simulink model "sedemo_timrecresample"  (Simulink 7.5)
settings: Solver=ode45  StartTime=0.0  StopTime=inf  MaxStep=1/(10*D*Fsymbol)  RelTol=1e-3
PreLoadFcn:
  | Fsymbol=1e6;
  | D=8;  % decimation / interpolation
  | Fdelay = 5;  % rrc filter delay
  | Alpha = 0.25;  % excess BW
  | rrc_coef=rcosine(1,D,'fir/sqrt',Alpha,Fdelay);
  | rrc_coef=rrc_coef/sum(rrc_coef);
  | Carrier_Freq = 21.4e6;
  | b3 = [1/6 -1/2  1/2 -1/6];
  | b2 = [1/2 -1    1/2  0];
  | b1 = [1/3  1/2 -1    1/6];
  | b0 = [0    1    0    0];
undefined symbols (not defined in the file or in its folder): dfilt, j, magnitude
libraries: dspsigops x29, simulink x13, dsparch4 x8, dspsrcs4 x4, dspbuff3 x2, simeventsinfo x1, simeventstranslate1 x1, dspmlti4 x1, commsink2 x1
CloseFcn:
  | clear Fsymbol D Fdelay Alpha rrc_coef Carrier_Freq b0 b1 b2 b3;
settings Model: Creator=The MathWorks Inc.  ExtModeAutoUpdateStatusClock=off
settings DataIOCC: SaveOutput=off  SignalLogging=off  SaveTime=off
settings OptimizationCC: InitFltsAndDblsToZero=on  EfficientMapNaN2IntZero=off
settings DebuggingCC: SignalResolutionControl=TryResolveAllWithWarning  MultiTaskDSMMsg=warning  MultiTaskCondExecSysMsg=none  SigSpecEnsureSampleTimeMsg=none  StrictBusMsg=None
settings RTWCC: IncludeERTFirstTime=on
settings SimEventsCC: propDiagAttribOutput=1  propDiagFcnCallOutput=1  propDiagStatOutput=0

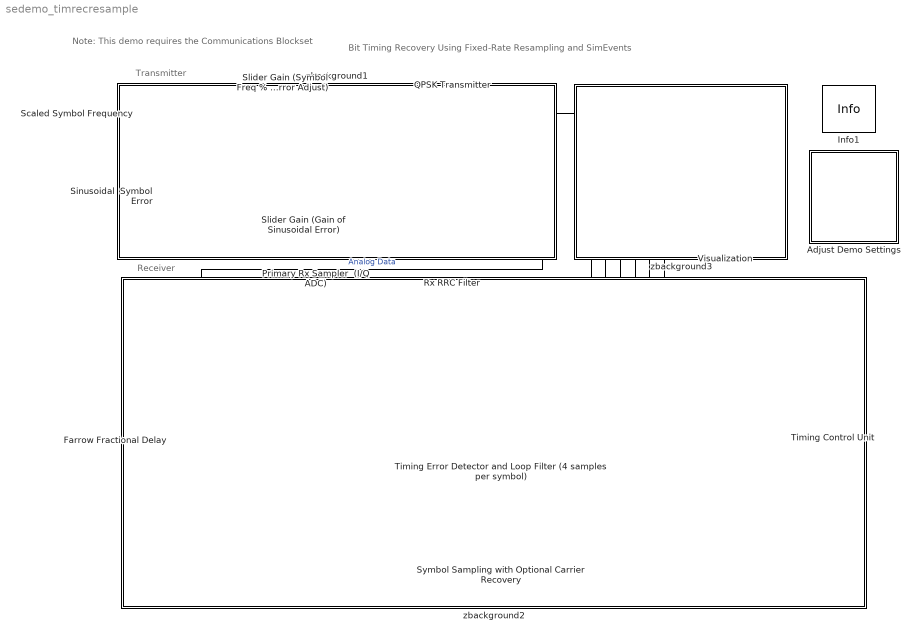
== system sedemo_timrecresample ==
  note: Bit Timing Recovery Using Fixed-Rate
      | Resampling and SimEvents
  note: Transmitter
  note: Receiver
  note: Note: This demo requires the
      | Communications Blockset
  Adjust Demo Settings : Subsystem  mask(Timing Recovery Demo Settings){enableTCU=on}
      mask prompts: enableTCU "Enable timing control"
      mask help:
      | Click on the 'Enable timing control' checkbox while the demo is running to enable and disable the timing control for the receiver.
      |
      | Note that you can also change the slider gain values for Symbol Frequency Percent Error and Gain of Sinusoidal Error while the demo is running.
      mask init:
      | set_param([bdroot '/Timing Control Unit/TCU_ON'],'Value',num2str(enableTCU));
      mask Display: disp('Timing\nRecovery\nDemo\nSettings');
  "Farrow Fractional Delay " : Subsystem
  Info1 : simeventsinfo/Info  SystemSampleTime=-1
  Primary Rx Sampler  (I/Q ADC) : ZeroOrderHold  SampleTime=1/(D*Fsymbol)
  QPSK Transmitter : Subsystem
  Rx RRC Filter : dspmlti4/FIR Decimation  DialogController=dspdialog.FIRDecimation  DialogControllerArgs=DataTag6  h=rrc_coef  D=2  filtStruct=Direct form  framing=Maintain input frame size  inputOffset=0  outputBufInitCond=0  roundingMode=Floor  overflowMode=off  FilterSource=Specify via dialog  FilterObject=Hm_firdecim
  Scaled Symbol Frequency : Constant  Value=(D*Fsymbol) / 100  OutDataType=sfix(16)  OutScaling=2^0
  Sinusoidal  Symbol Error : Sin  Amplitude=(D*Fsymbol) / 100  Bias=0  Frequency=(Fsymbol)*2*pi/1000  Phase=0  Samples=10  SampleTime=1e-5  Offset=0
  Slider Gain (Gain of Sinusoidal Error) : simulink/Math Operations/Slider Gain  SystemSampleTime=-1  low=0  gain=0.1  high=0.2
  Slider Gain (Symbol Freq % Error Adjust) : simulink/Math Operations/Slider Gain  SystemSampleTime=-1  low=-0.2  gain=0.02  high=0.2
  Symbol Sampling with Optional Carrier Recovery : Subsystem
  Timing Control Unit : Subsystem
  Timing Error Detector and Loop Filter (4 samples per symbol) : Subsystem
  Visualization : Subsystem
  zbackground1 : Subsystem
      mask Display: disp('')
  zbackground2 : Subsystem
      mask Display: disp('')
  zbackground3 : Subsystem
      mask Display: disp('')
  wires:
  Scaled Symbol Frequency/1 -> Slider Gain (Symbol Freq % Error Adjust)/1
  Slider Gain (Symbol Freq % Error Adjust)/1 -> QPSK Transmitter/1(Constant Sym Err)
  Slider Gain (Gain of Sinusoidal Error)/1 -> QPSK Transmitter/2(Sinusoidal Sym Err)
  Sinusoidal  Symbol Error/1 -> Slider Gain (Gain of Sinusoidal Error)/1
  QPSK Transmitter/1(Tx Sym Clk) -> Visualization/1(Tx Sym Clk)
  QPSK Transmitter/2(Tx Data) -> Primary Rx Sampler  (I/Q ADC)/1  "Analog Data"
  "Farrow Fractional Delay "/1(X(n-(1-u))) -> Timing Error Detector and Loop Filter (4 samples per symbol)/2(I/Q In), Symbol Sampling with Optional Carrier Recovery/2(Data)
  Primary Rx Sampler  (I/Q ADC)/1 -> Rx RRC Filter/1
  Rx RRC Filter/1 -> "Farrow Fractional Delay "/1(X(n))
  Timing Control Unit/1(Symbol Clk) -> Timing Error Detector and Loop Filter (4 samples per symbol)/1(Symbol Clk), Symbol Sampling with Optional Carrier Recovery/1(Symbol Clk), Visualization/2(Rx Rec Sym Clk)
  Timing Control Unit/2(Delay Ctrl) -> "Farrow Fractional Delay "/2(u), Visualization/7(Frac Dly Ctrl)
  Timing Error Detector and Loop Filter (4 samples per symbol)/2(Timing Ctrl) -> Timing Control Unit/1(Ctrl In), Visualization/4(TCU Ctrl)
  Timing Error Detector and Loop Filter (4 samples per symbol)/1(Timing Err) -> Visualization/3(Timing Err)
  Symbol Sampling with Optional Carrier Recovery/1(Delayed Clk) -> Visualization/5(Delayed Clk)
  Symbol Sampling with Optional Carrier Recovery/2(Symbol) -> Visualization/6(Rx Symbol)

== system sedemo_timrecresample/Adjust Demo Settings ==

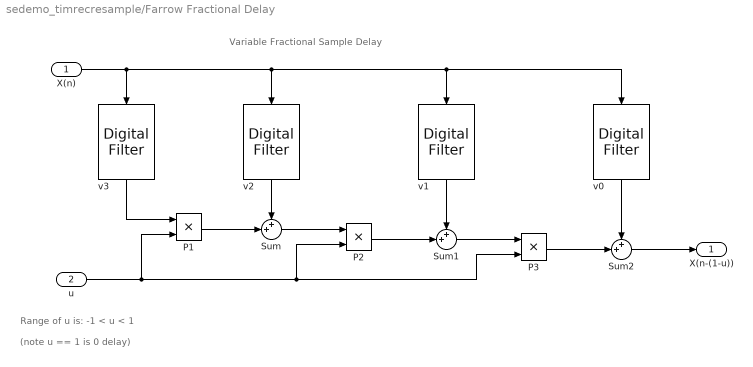
== system sedemo_timrecresample/Farrow Fractional Delay  ==
  note: Range of u is: -1 < u < 1
  note: Variable Fractional Sample Delay
  note: (note u == 1 is 0 delay)
  X(n) : Inport  OutDataType=sfix(16)  OutScaling=2^0
  u : Inport  Port=2  OutDataType=sfix(16)  OutScaling=2^0
  P1 : Product  OutDataType=sfix(16)  OutScaling=2^0  SaturateOnIntegerOverflow=on  OutDataTypeStr=Inherit: Same as first input
  P2 : Product  OutDataType=sfix(16)  OutScaling=2^0  SaturateOnIntegerOverflow=on  OutDataTypeStr=Inherit: Same as first input
  P3 : Product  OutDataType=sfix(16)  OutScaling=2^0  SaturateOnIntegerOverflow=on  OutDataTypeStr=Inherit: Same as first input
  Sum : Sum  Inputs=++|  OutDataType=sfix(16)  OutScaling=2^0  SaturateOnIntegerOverflow=on
  Sum1 : Sum  Inputs=++|  OutDataType=sfix(16)  OutScaling=2^0  SaturateOnIntegerOverflow=on
  Sum2 : Sum  Inputs=++|  OutDataType=sfix(16)  OutScaling=2^0  SaturateOnIntegerOverflow=on
  v0 : dsparch4/Digital Filter  DialogController=dspdialog.DigitalFilter  DialogControllerArgs=DataTag0  TypePopup=FIR (all zeros)  IIRFiltStruct=Direct form II transposed  AllPoleFiltStruct=Direct form  FIRFiltStruct=Direct form  CoeffSource=Specify via dialog  NumCoeffs=b0  DenCoeffs=[1 0.1]  BiQuadCoeffs=[1 0.3 0.4 1 0.1 0.2]  LatticeCoeffs=[0.2 0.4]  denIgnore=on  FiltPerSampPopup=One filter per frame  IC=0  ICnum=0  ICden=0  roundingMode=Floor  overflowMode=off  ScaleValues=1  scaleValueFracLength=14  stageInFracLength=15  stageOutFracLength=15  FilterSource=Specify via dialog  dfiltObjectName=dfilt.dffir([1 2 1])
  v1 : dsparch4/Digital Filter  DialogController=dspdialog.DigitalFilter  DialogControllerArgs=DataTag1  TypePopup=FIR (all zeros)  IIRFiltStruct=Direct form II transposed  AllPoleFiltStruct=Direct form  FIRFiltStruct=Direct form  CoeffSource=Specify via dialog  NumCoeffs=b1  DenCoeffs=[1 0.1]  BiQuadCoeffs=[1 0.3 0.4 1 0.1 0.2]  LatticeCoeffs=[0.2 0.4]  denIgnore=on  FiltPerSampPopup=One filter per frame  IC=0  ICnum=0  ICden=0  roundingMode=Floor  overflowMode=off  ScaleValues=1  scaleValueFracLength=14  stageInFracLength=15  stageOutFracLength=15  FilterSource=Specify via dialog  dfiltObjectName=dfilt.dffir([1 2 1])
  v2 : dsparch4/Digital Filter  DialogController=dspdialog.DigitalFilter  DialogControllerArgs=DataTag2  TypePopup=FIR (all zeros)  IIRFiltStruct=Direct form II transposed  AllPoleFiltStruct=Direct form  FIRFiltStruct=Direct form  CoeffSource=Specify via dialog  NumCoeffs=b2  DenCoeffs=[1 0.1]  BiQuadCoeffs=[1 0.3 0.4 1 0.1 0.2]  LatticeCoeffs=[0.2 0.4]  denIgnore=on  FiltPerSampPopup=One filter per frame  IC=0  ICnum=0  ICden=0  roundingMode=Floor  overflowMode=off  ScaleValues=1  scaleValueFracLength=14  stageInFracLength=15  stageOutFracLength=15  FilterSource=Specify via dialog  dfiltObjectName=dfilt.dffir([1 2 1])
  v3 : dsparch4/Digital Filter  DialogController=dspdialog.DigitalFilter  DialogControllerArgs=DataTag3  TypePopup=FIR (all zeros)  IIRFiltStruct=Direct form II transposed  AllPoleFiltStruct=Direct form  FIRFiltStruct=Direct form  CoeffSource=Specify via dialog  NumCoeffs=b3  DenCoeffs=[1 0.1]  BiQuadCoeffs=[1 0.3 0.4 1 0.1 0.2]  LatticeCoeffs=[0.2 0.4]  denIgnore=on  FiltPerSampPopup=One filter per frame  IC=0  ICnum=0  ICden=0  roundingMode=Floor  overflowMode=off  ScaleValues=1  scaleValueFracLength=14  stageInFracLength=15  stageOutFracLength=15  FilterSource=Specify via dialog  dfiltObjectName=dfilt.dffir([1 2 1])
  X(n-(1-u)) : Outport  OutDataType=sfix(16)  OutScaling=2^0
  wires:
  Sum2/1 -> X(n-(1-u))/1
  u/1 -> P3/2, P2/2, P1/2
  X(n)/1 -> v3/1, v2/1, v1/1, v0/1
  v0/1 -> Sum2/1
  v1/1 -> Sum1/1
  v2/1 -> Sum/1
  v3/1 -> P1/1
  P1/1 -> Sum/2
  Sum/1 -> P2/1
  P2/1 -> Sum1/2
  Sum1/1 -> P3/1
  P3/1 -> Sum2/2

== system sedemo_timrecresample/QPSK Transmitter ==
  note: 1/Ts=D*Fsymbol
  Constant Sym Err : Inport  OutDataType=sfix(16)  OutScaling=2^0
  Sinusoidal Sym Err : Inport  Port=2  OutDataType=sfix(16)  OutScaling=2^0
  Carrier Offset and Conversion to Continuous Time : Subsystem
  DES Voltage Controlled  Sample Rate : Subsystem
  Variable Rate Symbol Generator : Subsystem  TreatAsAtomicUnit=on
      settings: PropExecContextOutsideSubsystem=on
  Tx Sym Clk : Outport  OutDataType=sfix(16)  OutScaling=2^0
  Tx Data : Outport  Port=2  OutDataType=sfix(16)  OutScaling=2^0
  wires:
  Variable Rate Symbol Generator/1(RRC'd Symbols) -> Carrier Offset and Conversion to Continuous Time/1(Data)
  Carrier Offset and Conversion to Continuous Time/1(I/Q Out) -> Tx Data/1  "Baseband Continuous-Time Data"
  Sinusoidal Sym Err/1 -> DES Voltage Controlled  Sample Rate/2(Sinusoidal Error)
  Constant Sym Err/1 -> DES Voltage Controlled  Sample Rate/1(Constant Error)
  Variable Rate Symbol Generator/2(Symbol Clk) -> Tx Sym Clk/1  "Symbol Clock"
  DES Voltage Controlled  Sample Rate/1(Out1) -> Variable Rate Symbol Generator/Trigger

== system sedemo_timrecresample/Symbol Sampling with Optional Carrier Recovery ==
  note: Subsequent processing (demodulation, error correction, symbol to bit mapping, etc.)
      | may be placed inside the Symbol Sampler block.
  Symbol Clk : Inport  OutDataType=sfix(16)  OutScaling=2^0
  Data : Inport  Port=2  OutDataType=sfix(16)  OutScaling=2^0
  Carrier_Rec_ON : Constant  Value=0  OutDataTypeMode=boolean  OutDataType=sfix(16)  OutScaling=2^0  OutDataTypeStr=boolean
  Delay : dspsigops/Delay  dly_unit=Samples  delay=2  ic_detail=off  dif_ic_for_ch=off  dif_ic_for_dly=off  ic=0  reset_popup=None
  Symbol Sampler : Subsystem  TreatAsAtomicUnit=on
  Delayed Clk : Outport  OutDataType=sfix(16)  OutScaling=2^0
  Symbol : Outport  Port=2  OutDataType=sfix(16)  OutScaling=2^0
  wires:
  Delay/1 -> Delayed Clk/1, Symbol Sampler/Enable
  Symbol Clk/1 -> Delay/1
  Data/1 -> Symbol Sampler/1(In1)
  Symbol Sampler/1(Out1) -> Symbol/1
  Carrier_Rec_ON/1 -> Symbol Sampler/2(Carrier Recovery ON)

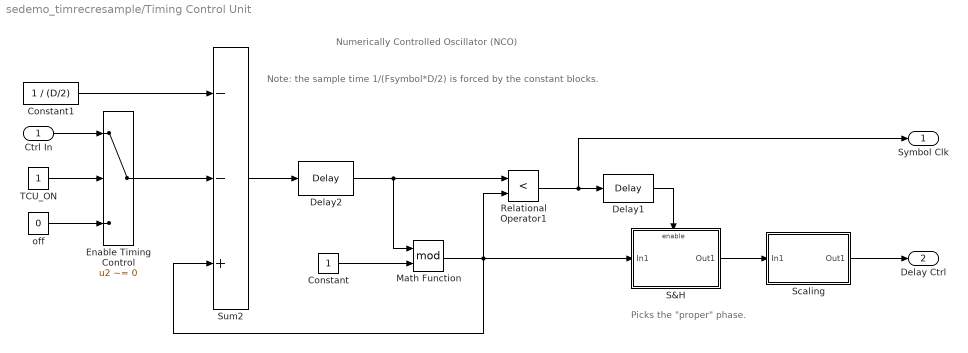
== system sedemo_timrecresample/Timing Control Unit ==
  note: Note:  the sample time 1/(Fsymbol*D/2)
      | is forced by the constant blocks.
  note: Numerically Controlled Oscillator (NCO)
  note: Picks the "proper" phase.
  Ctrl In : Inport  OutDataType=sfix(16)  OutScaling=2^0
  Constant : Constant  OutDataType=sfix(16)  OutScaling=2^0  OutDataTypeStr=Inherit: Inherit via back propagation  SampleTime=1/(Fsymbol*D/2)
  Constant1 : Constant  Value=1 / (D/2)  OutDataType=sfix(16)  OutScaling=2^0  OutDataTypeStr=Inherit: Inherit via back propagation  SampleTime=1/(Fsymbol*D/2)
  Delay1 : dspsigops/Delay  dly_unit=Samples  delay=1  ic_detail=off  dif_ic_for_ch=off  dif_ic_for_dly=off  ic=0  reset_popup=None
  Delay2 : dspsigops/Delay  dly_unit=Samples  delay=1  ic_detail=on  dif_ic_for_ch=off  dif_ic_for_dly=off  ic=0  reset_popup=None
  Enable Timing Control : Switch  Criteria=u2 ~= 0  OutDataType=sfix(16)  OutScaling=2^0
  Math Function : Math  Operator=mod  OutDataType=sfix(16)  OutScaling=2^0  SaturateOnIntegerOverflow=on
  Relational Operator1 : RelationalOperator  Operator=<  LogicOutDataTypeMode=boolean  LogicDataType=double(64)  OutDataTypeStr=boolean
  "S&H " : Subsystem  TreatAsAtomicUnit=on
  Scaling : Subsystem
  Sum2 : Sum  Inputs=--+  OutDataType=sfix(16)  OutScaling=2^0  SaturateOnIntegerOverflow=on  InputSameDT=on  OutDataTypeStr=Inherit: Same as first input
  TCU_ON : Constant  OutDataTypeMode=boolean  OutDataType=sfix(16)  OutScaling=2^0  OutDataTypeStr=boolean
  off : Constant  Value=0  OutDataType=sfix(16)  OutScaling=2^0
  Symbol Clk : Outport  OutDataType=sfix(16)  OutScaling=2^0
  Delay Ctrl : Outport  Port=2  OutDataType=sfix(16)  OutScaling=2^0
  wires:
  Delay2/1 -> Math Function/1, Relational Operator1/1
  Constant/1 -> Math Function/2
  Sum2/1 -> Delay2/1
  Constant1/1 -> Sum2/1
  Math Function/1 -> Sum2/3, Relational Operator1/2, "S&H "/1(In1)
  Relational Operator1/1 -> Delay1/1, Symbol Clk/1
  Delay1/1 -> "S&H "/Enable
  "S&H "/1(Out1) -> Scaling/1(In1)
  Scaling/1(Out1) -> Delay Ctrl/1
  TCU_ON/1 -> Enable Timing Control/2
  off/1 -> Enable Timing Control/3
  Ctrl In/1 -> Enable Timing Control/1
  Enable Timing Control/1 -> Sum2/2

== system sedemo_timrecresample/Timing Error Detector and Loop Filter (4 samples per symbol) ==
  note: H. Meyer et. al. Digital Communications Receivers, chapter 5.4, pp 291
  Symbol Clk : Inport  OutDataType=sfix(16)  OutScaling=2^0
  I/Q In : Inport  Port=2  OutDataType=sfix(16)  OutScaling=2^0
  Mag Sq + Delays : Subsystem
  Timing Error Detector : Subsystem  TreatAsAtomicUnit=on
  Timing Err : Outport  OutDataType=sfix(16)  OutScaling=2^0
  Timing Ctrl : Outport  Port=2  OutDataType=sfix(16)  OutScaling=2^0
  wires:
  Mag Sq + Delays/1(MagSq(u[n-1])) -> Timing Error Detector/1(In1)
  Mag Sq + Delays/2(MagSq(u[n-3])) -> Timing Error Detector/2(In2)
  Mag Sq + Delays/3(MagSq(u[n-2])) -> Timing Error Detector/3(In3)
  Mag Sq + Delays/4(MagSq(u[n])) -> Timing Error Detector/4(In4)
  I/Q In/1 -> Mag Sq + Delays/1(In1)
  Timing Error Detector/1(Error) -> Timing Err/1
  Timing Error Detector/2(Cntrl) -> Timing Ctrl/1
  Symbol Clk/1 -> Timing Error Detector/Enable

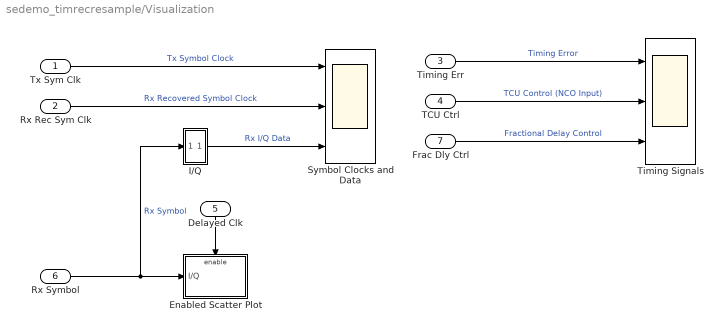
== system sedemo_timrecresample/Visualization ==
  Tx Sym Clk : Inport  OutDataType=sfix(16)  OutScaling=2^0
  Rx Rec Sym Clk : Inport  Port=2  OutDataType=sfix(16)  OutScaling=2^0
  Timing Err : Inport  Port=3  OutDataType=sfix(16)  OutScaling=2^0
  TCU Ctrl : Inport  Port=4  OutDataType=sfix(16)  OutScaling=2^0
  Delayed Clk : Inport  Port=5  OutDataType=sfix(16)  OutScaling=2^0
  Rx Symbol : Inport  Port=6  OutDataType=sfix(16)  OutScaling=2^0
  Frac Dly Ctrl : Inport  Port=7  OutDataType=sfix(16)  OutScaling=2^0
  Enabled Scatter Plot : Subsystem  TreatAsAtomicUnit=on
  I/Q : Subsystem
      mask Display: disp('')
  Symbol Clocks and Data : Scope  NumInputPorts=3
      settings: TimeRange=2e-06  YMin=-0.1~-0.1~-1.5  YMax=1.1~1.1~1.5
  Timing Signals : Scope  NumInputPorts=3
      settings: TimeRange=0.0002  YMin=-0.2~-0.001~-0.1  YMax=0.2~0.001~1.1  MaxDataPoints=50000
  wires:
  Rx Symbol/1 -> I/Q/1(cmplx), Enabled Scatter Plot/1(I/Q)  "Rx Symbol"
  I/Q/1(2x real) -> Symbol Clocks and Data/3  "Rx I/Q Data"
  Tx Sym Clk/1 -> Symbol Clocks and Data/1  "Tx Symbol Clock"
  Rx Rec Sym Clk/1 -> Symbol Clocks and Data/2  "Rx Recovered Symbol Clock"
  Timing Err/1 -> Timing Signals/1  "Timing Error"
  TCU Ctrl/1 -> Timing Signals/2  "TCU Control (NCO Input)"
  Frac Dly Ctrl/1 -> Timing Signals/3  "Fractional Delay Control"
  Delayed Clk/1 -> Enabled Scatter Plot/Enable

== system sedemo_timrecresample/zbackground1 ==

== system sedemo_timrecresample/zbackground2 ==

== system sedemo_timrecresample/zbackground3 ==

== system sedemo_timrecresample/QPSK Transmitter/Carrier Offset and Conversion to Continuous Time ==
  Data : Inport  OutDataType=sfix(16)  OutScaling=2^0
  Bessel LPF : Subsystem
  I/Q Out : Outport  OutDataType=sfix(16)  OutScaling=2^0
  wires:
  Data/1 -> Bessel LPF/1(In1)
  Bessel LPF/1(Out1) -> I/Q Out/1

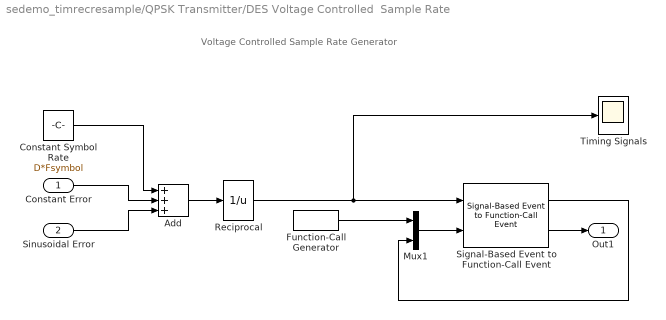
== system sedemo_timrecresample/QPSK Transmitter/DES Voltage Controlled  Sample Rate ==
  note: Voltage Controlled Sample Rate Generator
  Constant Error : Inport  OutDataType=sfix(16)  OutScaling=2^0
  Sinusoidal Error : Inport  Port=2  OutDataType=sfix(16)  OutScaling=2^0
  Add : Sum  Inputs=+++  OutDataType=sfix(16)  OutScaling=2^-10
  Constant Symbol Rate : Constant  Value=D*Fsymbol  OutDataType=sfix(16)  OutScaling=2^0
  Function-Call Generator : simulink/Ports & Subsystems/Function-Call Generator  sample_time=10000  numberOfIterations=1
  Mux1 : Mux  Inputs=2
  Reciprocal : Math  Operator=reciprocal  OutDataType=sfix(16)  OutScaling=2^0  SaturateOnIntegerOverflow=on
  Signal-Based Event to Function-Call Event : simeventstranslate1/Signal-Based Event to Function-Call Event  Priority=1  SystemSampleTime=-1  GenerateFunctionCallUpon=Function call from port fcn  SignalEdgeOption=Rising  EnableE1Port=off  EnableF2Port=on  EnableE2Port=off  SpecifyEventPriority=on  PriorityFunctionCall=200  FunctionCallDelayFrom=Signal port t  DelayFunctionCall=0  StatNumberF1Calls=Off  StatNumberF2Calls=Off  MaskBlockType=none
  Timing Signals : Scope
      settings: TimeRange=0.0006000000000000001  YMin=1.245e-007  YMax=1.27e-007  SaveName=ScopeData3  MaxDataPoints=50000
  Out1 : Outport  OutDataType=sfix(16)  OutScaling=2^0
  wires:
  Mux1/1 -> Signal-Based Event to Function-Call Event/2
  Function-Call Generator/1 -> Mux1/1
  Constant Symbol Rate/1 -> Add/1
  Add/1 -> Reciprocal/1
  Signal-Based Event to Function-Call Event/2 -> Out1/1
  Constant Error/1 -> Add/2
  Sinusoidal Error/1 -> Add/3
  Reciprocal/1 -> Signal-Based Event to Function-Call Event/1, Timing Signals/1
  Signal-Based Event to Function-Call Event/1 -> Mux1/2

== system sedemo_timrecresample/QPSK Transmitter/Variable Rate Symbol Generator ==
  note: Replace held value
      |  with zeros
      |  for proper interpolation.
  function : TriggerPort  TriggerType=function-call
  Complex Zero : Constant  Value=0+j*eps  OutDataType=sfix(16)  OutScaling=2^0
  Divide by D CLK : Subsystem  TreatAsAtomicUnit=on  mask(Pulse Divider){div=D, ph=2}
      mask prompts: div "Modulo:"; ph "Initial Phase Delay (cycles):"
  Gain : Gain  Gain=D  ParameterDataType=sfix(16)  ParameterScaling=2^0  OutDataType=sfix(16)  OutScaling=2^0
  Integer Delay : simulink/Discrete/Integer Delay  vinit=0.0  samptime=-1  NumDelays=6
  RRC Interpolating Filter : dsparch4/Digital Filter  DialogController=dspdialog.DigitalFilter  DialogControllerArgs=DataTag5  TypePopup=FIR (all zeros)  IIRFiltStruct=Direct form II transposed  AllPoleFiltStruct=Direct form  FIRFiltStruct=Direct form  CoeffSource=Specify via dialog  NumCoeffs=rrc_coef  DenCoeffs=[1 0.1]  BiQuadCoeffs=[1 0.3 0.4 1 0.1 0.2]  LatticeCoeffs=[0.2 0.4]  denIgnore=on  FiltPerSampPopup=One filter per frame  IC=0  ICnum=0  ICden=0  roundingMode=Floor  overflowMode=off  ScaleValues=1  scaleValueFracLength=14  stageInFracLength=15  stageOutFracLength=15  FilterSource=Specify via dialog  dfiltObjectName=dfilt.dffir([1 2 1])
  Switch : Switch  Threshold=.5  OutDataType=sfix(16)  OutScaling=2^0
  Symbol Gen : Subsystem  TreatAsAtomicUnit=on
  RRC'd Symbols : Outport  OutDataType=sfix(16)  OutScaling=2^0
  Symbol Clk : Outport  Port=2  OutDataType=sfix(16)  OutScaling=2^0
  wires:
  Divide by D CLK/1(" ") -> Symbol Gen/Trigger, Switch/2, Symbol Clk/1
  Symbol Gen/1(Out1) -> Switch/1
  Complex Zero/1 -> Switch/3
  Gain/1 -> Integer Delay/1
  RRC Interpolating Filter/1 -> RRC'd Symbols/1
  Switch/1 -> Gain/1
  Integer Delay/1 -> RRC Interpolating Filter/1

== system sedemo_timrecresample/Symbol Sampling with Optional Carrier Recovery/Symbol Sampler ==
  In1 : Inport  OutDataType=sfix(16)  OutScaling=2^0
  Carrier Recovery ON : Inport  Port=2  OutDataType=sfix(16)  OutScaling=2^0
  Enable : EnablePort
  Carrier Recovery : Subsystem  TreatAsAtomicUnit=on
  Switch : Switch  Threshold=.5  OutDataType=sfix(16)  OutScaling=2^0
  Out1 : Outport  OutDataType=sfix(16)  OutScaling=2^0  OutputWhenDisabled=reset  InitialOutput=0
  wires:
  Carrier Recovery ON/1 -> Carrier Recovery/Enable, Switch/2
  In1/1 -> Carrier Recovery/1(I/Q In), Switch/3
  Switch/1 -> Out1/1
  Carrier Recovery/1(Derotated I/Q Out) -> Switch/1

== system sedemo_timrecresample/Timing Control Unit/S&H  ==
  In1 : Inport  OutDataType=sfix(16)  OutScaling=2^0
  Enable : EnablePort
  Out1 : Outport  OutDataType=sfix(16)  OutScaling=2^0
  wires:
  In1/1 -> Out1/1

== system sedemo_timrecresample/Timing Control Unit/Scaling ==
  note: maps phase ramp of 0.5 to 0.75 to output of 0 to 1
  In1 : Inport  OutDataType=sfix(16)  OutScaling=2^0
  Add : Sum  OutDataType=sfix(16)  OutScaling=2^-10
  Gain2 : Gain  Gain=4  ParameterDataType=sfix(16)  ParameterScaling=2^0  OutDataType=sfix(16)  OutScaling=2^0
  k5 : Constant  Value=-2  OutDataType=sfix(16)  OutScaling=2^0  SampleTime=1/(Fsymbol*D/2)
  Out1 : Outport  OutDataType=sfix(16)  OutScaling=2^0
  wires:
  Add/1 -> Out1/1
  In1/1 -> Gain2/1
  k5/1 -> Add/2
  Gain2/1 -> Add/1

== system sedemo_timrecresample/Timing Error Detector and Loop Filter (4 samples per symbol)/Mag Sq + Delays ==
  note: Taking the mag squared makes this symbol timing detector impervious to carrier frequency shift.
      | Therefore, the simpler job of carrier recovery can be done after symbol retiming.
  In1 : Inport  OutDataType=sfix(16)  OutScaling=2^0
  Delay1 : dspsigops/Delay  dly_unit=Samples  delay=1  ic_detail=off  dif_ic_for_ch=off  dif_ic_for_dly=off  ic=0  reset_popup=None
  Delay2 : dspsigops/Delay  dly_unit=Samples  delay=1  ic_detail=off  dif_ic_for_ch=off  dif_ic_for_dly=off  ic=0  reset_popup=None
  Delay3 : dspsigops/Delay  dly_unit=Samples  delay=1  ic_detail=off  dif_ic_for_ch=off  dif_ic_for_dly=off  ic=0  reset_popup=None
  Math Function : Math  Operator=magnitude^2  OutDataType=sfix(16)  OutScaling=2^0  SaturateOnIntegerOverflow=on
  MagSq(u[n-1]) : Outport  OutDataType=sfix(16)  OutScaling=2^0
  MagSq(u[n-3]) : Outport  Port=2  OutDataType=sfix(16)  OutScaling=2^0
  MagSq(u[n-2]) : Outport  Port=3  OutDataType=sfix(16)  OutScaling=2^0
  MagSq(u[n]) : Outport  Port=4  OutDataType=sfix(16)  OutScaling=2^0
  wires:
  In1/1 -> Math Function/1
  Math Function/1 -> Delay1/1, MagSq(u[n])/1
  Delay1/1 -> Delay2/1, MagSq(u[n-1])/1
  Delay2/1 -> Delay3/1, MagSq(u[n-2])/1
  Delay3/1 -> MagSq(u[n-3])/1

== system sedemo_timrecresample/Timing Error Detector and Loop Filter (4 samples per symbol)/Timing Error Detector ==
  note: update once per symbol
  note: 4 samples per symbol are required
      | for this timing error estimator.
  In1 : Inport  OutDataType=sfix(16)  OutScaling=2^0
  In2 : Inport  Port=2  OutDataType=sfix(16)  OutScaling=2^0
  In3 : Inport  Port=3  OutDataType=sfix(16)  OutScaling=2^0
  In4 : Inport  Port=4  OutDataType=sfix(16)  OutScaling=2^0
  Enable : EnablePort
  "Loop Filter " : Subsystem  TreatAsAtomicUnit=on
  Timing Error : Subsystem
  Error : Outport  OutDataType=sfix(16)  OutScaling=2^0
  Cntrl : Outport  Port=2  OutDataType=sfix(16)  OutScaling=2^0
  wires:
  Timing Error/1(Out1) -> "Loop Filter "/1(In1), Error/1
  In1/1 -> Timing Error/1(In1)
  In2/1 -> Timing Error/2(In2)
  In3/1 -> Timing Error/3(In3)
  In4/1 -> Timing Error/4(In4)
  "Loop Filter "/1(Out1) -> Cntrl/1

== system sedemo_timrecresample/Visualization/Enabled Scatter Plot ==
  note: You can add demodulator, FEC, etc.
      | in this enabled subsystem.
  I/Q : Inport  OutDataType=sfix(16)  OutScaling=2^0
  Enable : EnablePort
  Discrete-Time Scatter Plot Scope2 : commsink2/Discrete-Time Scatter Plot Scope  Tag=ScatterPlot  SystemSampleTime=-1  sampPerSymb=1  offsetEye=0  numTraces=80  numNewFrames=7  LineMarkers=.  LineColors=b  fading=on  render=on  AxisGrid=on  xMin=-1.5  xMax=1.5  yMin=-1.5  yMax=1.5  inphaseLabel=In-phase Amplitude  quadratureLabel=Quadrature Amplitude  openScopeAtSimStart=on  FrameNumber=off  FigPos=[546 39 317 317]  figTitle=Received Symbol  numLinesMax=8  block_type_=scatter
  wires:
  I/Q/1 -> Discrete-Time Scatter Plot Scope2/1

== system sedemo_timrecresample/Visualization/I/Q ==
  note: to visually align traces
  cmplx : Inport  OutDataType=sfix(16)  OutScaling=2^0
  Complex to Real-Imag : ComplexToRealImag
  Delay1 : dspsigops/Delay  dly_unit=Samples  delay=2  ic_detail=off  dif_ic_for_ch=off  dif_ic_for_dly=off  ic=0  reset_popup=None
  Mux : Mux  Inputs=2
  2x real : Outport  OutDataType=sfix(16)  OutScaling=2^0
  wires:
  Complex to Real-Imag/1 -> Mux/1
  Complex to Real-Imag/2 -> Mux/2
  cmplx/1 -> Complex to Real-Imag/1
  Mux/1 -> Delay1/1
  Delay1/1 -> 2x real/1

== system sedemo_timrecresample/QPSK Transmitter/Carrier Offset and Conversion to Continuous Time/Bessel LPF ==
  In1 : Inport  OutDataType=sfix(16)  OutScaling=2^0
  Analog Filter Design : dsparch4/Analog Filter Design  method=Bessel  filttype=Lowpass  N=8  Wlo=2*pi*D*Fsymbol*0.3  Whi=80  Rp=2  Rs=40
  Analog Filter Design1 : dsparch4/Analog Filter Design  method=Bessel  filttype=Lowpass  N=8  Wlo=2*pi*D*Fsymbol*0.3  Whi=80  Rp=2  Rs=40
  Complex to Real-Imag : ComplexToRealImag
  Real-Imag to Complex1 : RealImagToComplex
  Out1 : Outport  OutDataType=sfix(16)  OutScaling=2^0
  wires:
  In1/1 -> Complex to Real-Imag/1
  Real-Imag to Complex1/1 -> Out1/1
  Analog Filter Design1/1 -> Real-Imag to Complex1/2
  Analog Filter Design/1 -> Real-Imag to Complex1/1
  Complex to Real-Imag/2 -> Analog Filter Design1/1
  Complex to Real-Imag/1 -> Analog Filter Design/1

== system sedemo_timrecresample/QPSK Transmitter/Variable Rate Symbol Generator/Divide by D CLK ==
  Constant1 : Constant  Value=div  OutDataType=sfix(16)  OutScaling=2^0
  Constant2 : Constant  OutDataType=sfix(16)  OutScaling=2^0
  Fcn4 : Fcn  Expr=u<1
  Math Function : Math  Operator=mod  OutDataType=sfix(16)  OutScaling=2^0  SaturateOnIntegerOverflow=on
  Sum : Sum  Inputs=|++  OutDataType=sfix(16)  OutScaling=2^0  SaturateOnIntegerOverflow=on  InputSameDT=on  OutDataTypeStr=Inherit: Same as first input
  Unit Delay : UnitDelay  X0=div-ph  SampleTime=-1
  " " : Outport  OutDataType=sfix(16)  OutScaling=2^0
  wires:
  Fcn4/1 -> " "/1
  Constant1/1 -> Math Function/2
  Math Function/1 -> Fcn4/1, Sum/2
  Unit Delay/1 -> Math Function/1
  Constant2/1 -> Sum/1
  Sum/1 -> Unit Delay/1

== system sedemo_timrecresample/QPSK Transmitter/Variable Rate Symbol Generator/Symbol Gen ==
  Trigger : TriggerPort
  PN1 : Subsystem  mask(PN(10) Sequence [3,10]){}
      mask help: Pseudo Noise Sequence (M=2^10 - 1, Feedback[3,10])
      mask init:
      | [x,y]=commsrcsicon(5);
      mask Help: Maximal length pseudo-noise sequence with 10 memory elements.  Feedback is from taps 3 and 10.  Only the 10th tap is output.
      mask Display: plot(0,0,100,100,x,y);disp('PN Sequence ')
  QPSK : Subsystem
  Out1 : Outport  OutDataType=sfix(16)  OutScaling=2^0
  wires:
  PN1/1(Tap10) -> QPSK/1(In1)
  PN1/2(Tap2) -> QPSK/2(In2)
  QPSK/1(Out1) -> Out1/1

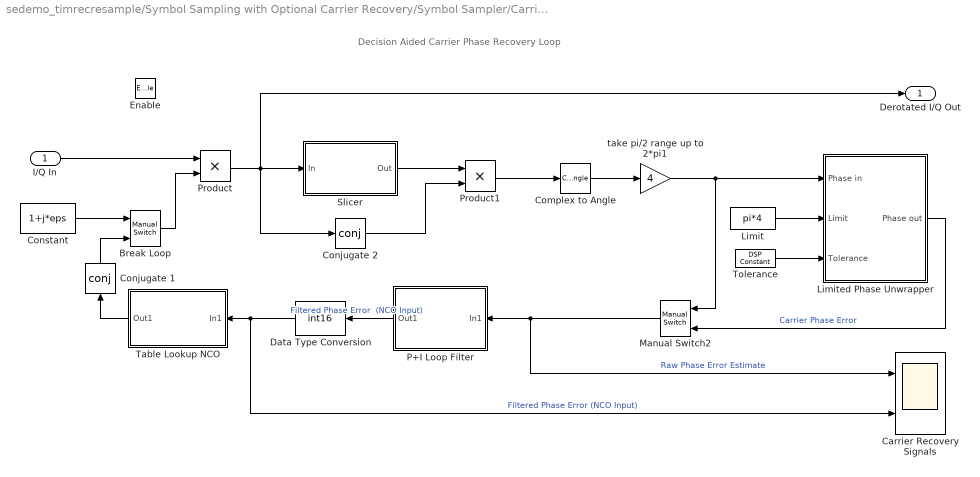
== system sedemo_timrecresample/Symbol Sampling with Optional Carrier Recovery/Symbol Sampler/Carrier Recovery ==
  note: Decision Aided Carrier Phase Recovery Loop
  I/Q In : Inport  OutDataType=sfix(16)  OutScaling=2^0
  Enable : EnablePort
  Break Loop : simulink/Signal Routing/Manual Switch  SystemSampleTime=-1  sw=0  action=0  varsize=off
  Carrier Recovery Signals : Scope  NumInputPorts=2
      settings: TimeRange=0.0002  YMin=-0.5~-10  YMax=0.5~10  SaveName=ScopeData2  MaxDataPoints=50000
  Complex to Angle : ComplexToMagnitudeAngle  Output=Angle
  Conjugate 1 : Math  Operator=conj  OutDataType=sfix(16)  OutScaling=2^0  SaturateOnIntegerOverflow=on
  Conjugate 2 : Math  Operator=conj  OutDataType=sfix(16)  OutScaling=2^0  SaturateOnIntegerOverflow=on
  Constant : Constant  Value=1+j*eps  OutDataType=sfix(16)  OutScaling=2^0
  Data Type Conversion : DataTypeConversion  OutDataTypeMode=int16  OutDataType=sfix(16)  OutScaling=2^0  OutDataTypeStr=int16  RndMeth=Nearest  SaturateOnIntegerOverflow=on
  Limit : Constant  Value=pi*4  VectorParams1D=off  OutDataType=sfix(16)  OutScaling=2^0
  Limited Phase Unwrapper : Subsystem
  Manual Switch2 : simulink/Signal Routing/Manual Switch  SystemSampleTime=-1  sw=0  action=0  varsize=off
  P+I Loop Filter : Subsystem
  Product : Product  OutDataType=sfix(16)  OutScaling=2^0  RndMeth=Zero
  Product1 : Product  OutDataType=sfix(16)  OutScaling=2^0  RndMeth=Zero
  Slicer : Subsystem
  Table Lookup NCO : Subsystem
  Tolerance : dspsrcs4/DSP Constant  SystemSampleTime=-1  Value=pi  SampleMode=Discrete  discreteOutput=Sample-based  continuousOutput=Sample-based  sampTime=inf  framePeriod=2  dataType=double  isSigned=on  wordLen=16  udDataType=sfix(16)  fracBitsMode=Best precision  numFracBits=15  InterpretAs1D=-inf  Ts=-inf  FramebasedOutput=-inf
      settings: additionalParams=on
  take pi/2 range up to 2*pi1 : Gain  Gain=4  ParameterDataType=sfix(16)  ParameterScaling=2^0  OutDataType=sfix(16)  OutScaling=2^0
  Derotated I/Q Out : Outport  OutDataType=sfix(16)  OutScaling=2^0
  wires:
  P+I Loop Filter/1(Out1) -> Data Type Conversion/1  "Filtered Phase Error  (NCO Input)"
  Table Lookup NCO/1(Out1) -> Conjugate 1/1
  Constant/1 -> Break Loop/1
  Conjugate 1/1 -> Break Loop/2
  Break Loop/1 -> Product/2
  Product1/1 -> Complex to Angle/1
  Conjugate 2/1 -> Product1/2
  Slicer/1(Out) -> Product1/1
  Product/1 -> Derotated I/Q Out/1, Conjugate 2/1, Slicer/1(In)
  I/Q In/1 -> Product/1
  Complex to Angle/1 -> take pi/2 range up to 2*pi1/1
  Limit/1 -> Limited Phase Unwrapper/2(Limit)
  Tolerance/1 -> Limited Phase Unwrapper/3(Tolerance)
  Limited Phase Unwrapper/1(Phase out) -> Manual Switch2/2  "Carrier Phase Error"
  Manual Switch2/1 -> P+I Loop Filter/1(In1), Carrier Recovery Signals/1  "Raw Phase Error Estimate"
  take pi/2 range up to 2*pi1/1 -> Limited Phase Unwrapper/1(Phase in), Manual Switch2/1
  Data Type Conversion/1 -> Table Lookup NCO/1(In1), Carrier Recovery Signals/2  "Filtered Phase Error (NCO Input)"

== system sedemo_timrecresample/Timing Error Detector and Loop Filter (4 samples per symbol)/Timing Error Detector/Loop Filter  ==
  note: Integrator
  note: PID Loop Filter
  In1 : Inport  OutDataType=sfix(16)  OutScaling=2^0
  Derivative : Gain  Gain=10  ParameterDataType=sfix(16)  ParameterScaling=2^0  OutDataType=sfix(16)  OutScaling=2^0
  Digital Filter : dsparch4/Digital Filter  DialogController=dspdialog.DigitalFilter  DialogControllerArgs=DataTag7  TypePopup=IIR (poles & zeros)  IIRFiltStruct=Direct form II transposed  AllPoleFiltStruct=Direct form  FIRFiltStruct=Direct form  CoeffSource=Specify via dialog  NumCoeffs=[.02]  DenCoeffs=[1 -1]  BiQuadCoeffs=[1 0.3 0.4 1 0.1 0.2]  LatticeCoeffs=[0.2 0.4]  denIgnore=on  FiltPerSampPopup=One filter per frame  IC=0  ICnum=0  ICden=0  roundingMode=Floor  overflowMode=off  ScaleValues=1  scaleValueFracLength=14  stageInFracLength=15  stageOutFracLength=15  FilterSource=Specify via dialog  dfiltObjectName=dfilt.dffir([1 2 1])
  Gain1 : Gain  Gain=-0.001  ParameterDataType=sfix(16)  ParameterScaling=2^0  OutDataType=sfix(16)  OutScaling=2^0
  Integer Delay : simulink/Discrete/Integer Delay  vinit=0.0  samptime=-1  NumDelays=5
  Proportional : Gain  Gain=5  ParameterDataType=sfix(16)  ParameterScaling=2^0  OutDataType=sfix(16)  OutScaling=2^0
  Smoothing Filter : DiscreteTransferFcn  Numerator=0.05  Denominator=[1 -0.95]  SampleTime=-1
  Sum1 : Sum  Inputs=+++  OutDataType=sfix(16)  OutScaling=2^0  SaturateOnIntegerOverflow=on  InputSameDT=on  OutDataTypeStr=Inherit: Same as first input
  Sum2 : Sum  Inputs=+-  OutDataType=sfix(16)  OutScaling=2^0  SaturateOnIntegerOverflow=on  InputSameDT=on  OutDataTypeStr=Inherit: Same as first input
  Out1 : Outport  OutDataType=sfix(16)  OutScaling=2^0
  wires:
  In1/1 -> Digital Filter/1, Smoothing Filter/1
  Digital Filter/1 -> Sum1/1
  Sum1/1 -> Gain1/1
  Integer Delay/1 -> Sum2/2
  Sum2/1 -> Derivative/1
  Proportional/1 -> Sum1/2
  Gain1/1 -> Out1/1
  Derivative/1 -> Sum1/3
  Smoothing Filter/1 -> Proportional/1, Integer Delay/1, Sum2/1

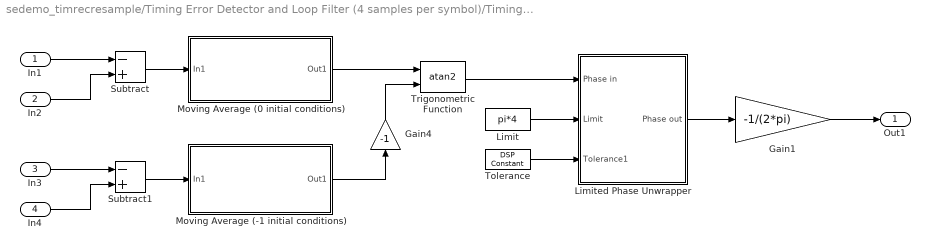
== system sedemo_timrecresample/Timing Error Detector and Loop Filter (4 samples per symbol)/Timing Error Detector/Timing Error ==
  In1 : Inport  OutDataType=sfix(16)  OutScaling=2^0
  In2 : Inport  Port=2  OutDataType=sfix(16)  OutScaling=2^0
  In3 : Inport  Port=3  OutDataType=sfix(16)  OutScaling=2^0
  In4 : Inport  Port=4  OutDataType=sfix(16)  OutScaling=2^0
  Gain1 : Gain  Gain=-1/(2*pi)  ParameterDataType=sfix(16)  ParameterScaling=2^0  OutDataType=sfix(16)  OutScaling=2^0
  Gain4 : Gain  Gain=-1  ParameterDataType=sfix(16)  ParameterScaling=2^0  OutDataType=sfix(16)  OutScaling=2^0
  Limit : Constant  Value=pi*4  VectorParams1D=off  OutDataType=sfix(16)  OutScaling=2^0
  Limited Phase Unwrapper : Subsystem
  Moving Average (-1 initial conditions) : Subsystem
  Moving Average (0 initial conditions) : Subsystem
  Subtract : Sum  Inputs=-+  OutDataType=sfix(16)  OutScaling=2^-10
  Subtract1 : Sum  Inputs=-+  OutDataType=sfix(16)  OutScaling=2^-10
  Tolerance : dspsrcs4/DSP Constant  SystemSampleTime=-1  Value=pi  SampleMode=Discrete  discreteOutput=Sample-based  continuousOutput=Sample-based  sampTime=inf  framePeriod=2  dataType=double  isSigned=on  wordLen=16  udDataType=sfix(16)  fracBitsMode=Best precision  numFracBits=15  InterpretAs1D=-inf  Ts=-inf  FramebasedOutput=-inf
      settings: additionalParams=on
  Trigonometric Function : Trigonometry  Operator=atan2
  Out1 : Outport  OutDataType=sfix(16)  OutScaling=2^0
  wires:
  In4/1 -> Subtract1/2
  In3/1 -> Subtract1/1
  In2/1 -> Subtract/2
  In1/1 -> Subtract/1
  Moving Average (-1 initial conditions)/1(Out1) -> Gain4/1
  Gain4/1 -> Trigonometric Function/2
  Limited Phase Unwrapper/1(Phase out) -> Gain1/1
  Gain1/1 -> Out1/1
  Subtract/1 -> Moving Average (0 initial conditions)/1(In1)
  Subtract1/1 -> Moving Average (-1 initial conditions)/1(In1)
  Trigonometric Function/1 -> Limited Phase Unwrapper/1(Phase in)
  Limit/1 -> Limited Phase Unwrapper/2(Limit)
  Tolerance/1 -> Limited Phase Unwrapper/3(Tolerance1)
  Moving Average (0 initial conditions)/1(Out1) -> Trigonometric Function/1

== system sedemo_timrecresample/QPSK Transmitter/Variable Rate Symbol Generator/Symbol Gen/PN1 ==
  Subsystem : Subsystem
  Subsystem1 : Subsystem
  Terminator : Terminator
  Terminator1 : Terminator
  Tap10 : Outport  OutDataType=sfix(16)  OutScaling=2^0  InitialOutput=0
  Tap2 : Outport  Port=2  OutDataType=sfix(16)  OutScaling=2^0  InitialOutput=0
  wires:
  Subsystem/1(Tap10) -> Tap10/1
  Subsystem1/2(Tap2) -> Tap2/1
  Subsystem/2(Tap2) -> Terminator/1
  Subsystem1/1(Tap10) -> Terminator1/1

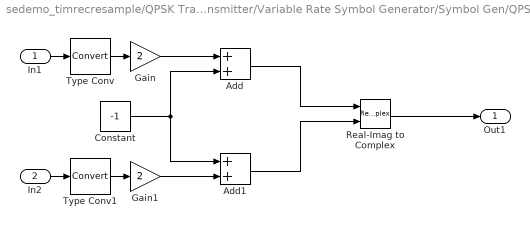
== system sedemo_timrecresample/QPSK Transmitter/Variable Rate Symbol Generator/Symbol Gen/QPSK ==
  In1 : Inport  OutDataType=sfix(16)  OutScaling=2^0
  In2 : Inport  Port=2  OutDataType=sfix(16)  OutScaling=2^0
  Add : Sum  OutDataType=sfix(16)  OutScaling=2^-10
  Add1 : Sum  OutDataType=sfix(16)  OutScaling=2^-10
  Constant : Constant  Value=-1  OutDataType=sfix(16)  OutScaling=2^0
  Gain : Gain  Gain=2  ParameterDataType=sfix(16)  ParameterScaling=2^0  OutDataType=sfix(16)  OutScaling=2^0
  Gain1 : Gain  Gain=2  ParameterDataType=sfix(16)  ParameterScaling=2^0  OutDataType=sfix(16)  OutScaling=2^0
  Real-Imag to Complex : RealImagToComplex
  Type Conv : DataTypeConversion  OutDataType=sfix(16)  OutScaling=2^0
  Type Conv1 : DataTypeConversion  OutDataType=sfix(16)  OutScaling=2^0
  Out1 : Outport  OutDataType=sfix(16)  OutScaling=2^0
  wires:
  Real-Imag to Complex/1 -> Out1/1
  In2/1 -> Type Conv1/1
  Add/1 -> Real-Imag to Complex/1
  In1/1 -> Type Conv/1
  Gain/1 -> Add/1
  Constant/1 -> Add/2, Add1/1
  Gain1/1 -> Add1/2
  Add1/1 -> Real-Imag to Complex/2
  Type Conv/1 -> Gain/1
  Type Conv1/1 -> Gain1/1

== system sedemo_timrecresample/Symbol Sampling with Optional Carrier Recovery/Symbol Sampler/Carrier Recovery/Limited Phase Unwrapper ==
  Phase in : Inport  OutDataType=sfix(16)  OutScaling=2^0
  Limit : Inport  Port=2  OutDataType=sfix(16)  OutScaling=2^0
  Tolerance : Inport  Port=3  OutDataType=sfix(16)  OutScaling=2^0
  Abs : Abs  OutDataType=sfix(16)  OutScaling=2^0  SaturateOnIntegerOverflow=on
  Delay : dspsigops/Delay  dly_unit=Samples  delay=1  ic_detail=off  dif_ic_for_ch=off  dif_ic_for_dly=off  ic=0  reset_popup=None
  N*2*pi accumulator : Subsystem  TreatAsAtomicUnit=on
  Relational Operator : RelationalOperator
  Sum : Sum  Inputs=|-+  OutDataType=sfix(16)  OutScaling=2^0  SaturateOnIntegerOverflow=on
  Sum1 : Sum  Inputs=|++  OutDataType=sfix(16)  OutScaling=2^0  SaturateOnIntegerOverflow=on
  Phase out : Outport  OutDataType=sfix(16)  OutScaling=2^0
  wires:
  Phase in/1 -> Sum1/1, Sum/2, Delay/1
  Delay/1 -> Sum/1
  Sum/1 -> Abs/1, N*2*pi accumulator/1(add_sub)
  Abs/1 -> Relational Operator/1
  Tolerance/1 -> Relational Operator/2
  Relational Operator/1 -> N*2*pi accumulator/Enable
  N*2*pi accumulator/1(K*2*pi) -> Sum1/2
  Sum1/1 -> Phase out/1
  Limit/1 -> N*2*pi accumulator/2(Limit)

== system sedemo_timrecresample/Symbol Sampling with Optional Carrier Recovery/Symbol Sampler/Carrier Recovery/P+I Loop Filter ==
  In1 : Inport  OutDataType=sfix(16)  OutScaling=2^0
  Add : Sum  OutDataType=sfix(16)  OutScaling=2^-10
  Add1 : Sum  OutDataType=sfix(16)  OutScaling=2^-10
  I gain : Gain  Gain=-.2  ParameterDataType=sfix(16)  ParameterScaling=2^0  OutDataType=sfix(16)  OutScaling=2^0
  Integer Delay : simulink/Discrete/Integer Delay  vinit=0.0  samptime=-1  NumDelays=1
  P gain : Gain  Gain=-2  ParameterDataType=sfix(16)  ParameterScaling=2^0  OutDataType=sfix(16)  OutScaling=2^0
  Saturation : Saturate  UpperLimit=60  LowerLimit=-60  OutDataType=sfix(16)  OutScaling=2^0
  Saturation1 : Saturate  UpperLimit=60  LowerLimit=-60  OutDataType=sfix(16)  OutScaling=2^0
  gain : Gain  Gain=5  ParameterDataType=sfix(16)  ParameterScaling=2^0  OutDataType=sfix(16)  OutScaling=2^0
  Out1 : Outport  OutDataType=sfix(16)  OutScaling=2^0
  wires:
  Add/1 -> Saturation1/1
  In1/1 -> gain/1
  I gain/1 -> Add1/1
  Integer Delay/1 -> Add1/2
  Add1/1 -> Add/2, Saturation/1
  P gain/1 -> Add/1
  gain/1 -> I gain/1, P gain/1
  Saturation/1 -> Integer Delay/1
  Saturation1/1 -> Out1/1

== system sedemo_timrecresample/Symbol Sampling with Optional Carrier Recovery/Symbol Sampler/Carrier Recovery/Slicer ==
  In : Inport  OutDataType=sfix(16)  OutScaling=2^0
  Complex to Real-Imag : ComplexToRealImag
  Gain1 : Gain  Gain=1/sqrt(2)  ParameterDataType=sfix(16)  ParameterScaling=2^0  OutDataType=sfix(16)  OutScaling=2^0
  Real-Imag to Complex : RealImagToComplex
  Sign : Signum
  Sign1 : Signum
  Out : Outport  OutDataType=sfix(16)  OutScaling=2^0
  wires:
  In/1 -> Complex to Real-Imag/1
  Complex to Real-Imag/1 -> Sign/1
  Complex to Real-Imag/2 -> Sign1/1
  Sign/1 -> Real-Imag to Complex/1
  Sign1/1 -> Real-Imag to Complex/2
  Real-Imag to Complex/1 -> Gain1/1
  Gain1/1 -> Out/1

== system sedemo_timrecresample/Symbol Sampling with Optional Carrier Recovery/Symbol Sampler/Carrier Recovery/Table Lookup NCO ==
  In1 : Inport  OutDataType=sfix(16)  OutScaling=2^0
  Add2 : Sum  OutDataType=sfix(16)  OutScaling=2^-10
  Constant1 : Constant  Value=(2^10)-1  OutDataType=sfix(16)  OutScaling=2^0
  Integer Delay1 : simulink/Discrete/Integer Delay  vinit=0.0  samptime=-1  NumDelays=1
  Math Function2 : Math  Operator=mod  OutDataType=sfix(16)  OutScaling=2^0  SaturateOnIntegerOverflow=on
  Real-Imag to Complex : RealImagToComplex
  cos : Lookup  InputValues=[0:1023]  Table=cos((0:1023)*2*pi/1024)  LookUpMeth=Use Input Below  OutDataType=sfix(16)  OutScaling=2^0
  sin : Lookup  InputValues=[0:1023]  Table=sin((0:1023)*2*pi/1024)  LookUpMeth=Use Input Below  OutDataType=sfix(16)  OutScaling=2^0
  Out1 : Outport  OutDataType=sfix(16)  OutScaling=2^0
  wires:
  cos/1 -> Real-Imag to Complex/1
  sin/1 -> Real-Imag to Complex/2
  Math Function2/1 -> Integer Delay1/1
  Real-Imag to Complex/1 -> Out1/1
  In1/1 -> Add2/1
  Constant1/1 -> Math Function2/2
  Add2/1 -> Math Function2/1
  Integer Delay1/1 -> cos/1, sin/1, Add2/2

== system sedemo_timrecresample/Timing Error Detector and Loop Filter (4 samples per symbol)/Timing Error Detector/Timing Error/Limited Phase Unwrapper ==
  Phase in : Inport  OutDataType=sfix(16)  OutScaling=2^0
  Limit : Inport  Port=2  OutDataType=sfix(16)  OutScaling=2^0
  Tolerance1 : Inport  Port=3  OutDataType=sfix(16)  OutScaling=2^0
  Abs : Abs  OutDataType=sfix(16)  OutScaling=2^0  SaturateOnIntegerOverflow=on
  Delay : dspsigops/Delay  dly_unit=Samples  delay=1  ic_detail=off  dif_ic_for_ch=off  dif_ic_for_dly=off  ic=0  reset_popup=None
  N*2*pi accumulator : Subsystem  TreatAsAtomicUnit=on
  Relational Operator : RelationalOperator
  Sum : Sum  Inputs=|-+  OutDataType=sfix(16)  OutScaling=2^0  SaturateOnIntegerOverflow=on
  Sum1 : Sum  Inputs=|++  OutDataType=sfix(16)  OutScaling=2^0  SaturateOnIntegerOverflow=on
  Phase out : Outport  OutDataType=sfix(16)  OutScaling=2^0
  wires:
  Phase in/1 -> Sum1/1, Sum/2, Delay/1
  Delay/1 -> Sum/1
  Sum/1 -> Abs/1, N*2*pi accumulator/1(add_sub)
  Abs/1 -> Relational Operator/1
  Tolerance1/1 -> Relational Operator/2
  Relational Operator/1 -> N*2*pi accumulator/Enable
  N*2*pi accumulator/1(K*2*pi) -> Sum1/2
  Sum1/1 -> Phase out/1
  Limit/1 -> N*2*pi accumulator/2(Limit)

== system sedemo_timrecresample/Timing Error Detector and Loop Filter (4 samples per symbol)/Timing Error Detector/Timing Error/Moving Average (-1 initial conditions) ==
  In1 : Inport  OutDataType=sfix(16)  OutScaling=2^0
  Delay Line1 : dspbuff3/Delay Line  siz=50  ic=-1  directfeed=on
  Frame Conversion1 : FrameConversion  OutFrame=Sample-based
  Sum of Elements1 : Sum  Inputs=+  OutDataType=sfix(16)  OutScaling=2^-10
  Out1 : Outport  OutDataType=sfix(16)  OutScaling=2^0
  wires:
  Delay Line1/1 -> Sum of Elements1/1
  Sum of Elements1/1 -> Frame Conversion1/1
  In1/1 -> Delay Line1/1
  Frame Conversion1/1 -> Out1/1

== system sedemo_timrecresample/Timing Error Detector and Loop Filter (4 samples per symbol)/Timing Error Detector/Timing Error/Moving Average (0 initial conditions) ==
  In1 : Inport  OutDataType=sfix(16)  OutScaling=2^0
  Delay Line : dspbuff3/Delay Line  siz=50  ic=0  directfeed=on
  Frame Conversion : FrameConversion  OutFrame=Sample-based
  Sum of Elements : Sum  Inputs=+  OutDataType=sfix(16)  OutScaling=2^-10
  Out1 : Outport  OutDataType=sfix(16)  OutScaling=2^0
  wires:
  Delay Line/1 -> Sum of Elements/1
  Sum of Elements/1 -> Frame Conversion/1
  In1/1 -> Delay Line/1
  Frame Conversion/1 -> Out1/1

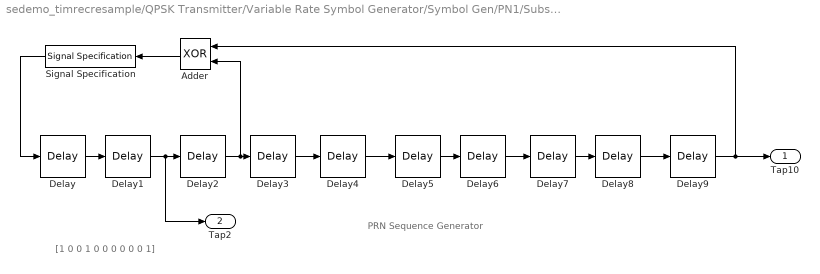
== system sedemo_timrecresample/QPSK Transmitter/Variable Rate Symbol Generator/Symbol Gen/PN1/Subsystem ==
  note: [1 0 0 1 0 0 0 0 0 0 1]
  note: PRN Sequence Generator
  Adder : Logic  Operator=XOR
  Delay{,3..8} (7 alike) : dspsigops/Delay  dly_unit=Samples  delay=1  ic_detail=on  dif_ic_for_ch=off  dif_ic_for_dly=off  ic=1  reset_popup=None
  Delay1 : dspsigops/Delay  dly_unit=Samples  delay=1  ic_detail=on  dif_ic_for_ch=off  dif_ic_for_dly=off  ic=0  reset_popup=None
  Delay2 : dspsigops/Delay  dly_unit=Samples  delay=1  ic_detail=on  dif_ic_for_ch=off  dif_ic_for_dly=off  ic=0  reset_popup=None
  Delay9 : dspsigops/Delay  dly_unit=Samples  delay=1  ic_detail=on  dif_ic_for_ch=off  dif_ic_for_dly=off  ic=0  reset_popup=None
  Signal Specification : SignalSpecification  OutDataType=sfix(16)  OutScaling=2^0
  Tap10 : Outport  OutDataType=sfix(16)  OutScaling=2^0  InitialOutput=0
  Tap2 : Outport  Port=2  OutDataType=sfix(16)  OutScaling=2^0  InitialOutput=0
  wires:
  Delay2/1 -> Adder/2, Delay3/1
  Adder/1 -> Signal Specification/1
  Delay8/1 -> Delay9/1
  Delay7/1 -> Delay8/1
  Delay6/1 -> Delay7/1
  Delay5/1 -> Delay6/1
  Delay4/1 -> Delay5/1
  Delay3/1 -> Delay4/1
  Delay1/1 -> Tap2/1, Delay2/1
  Delay/1 -> Delay1/1
  Delay9/1 -> Tap10/1, Adder/1
  Signal Specification/1 -> Delay/1

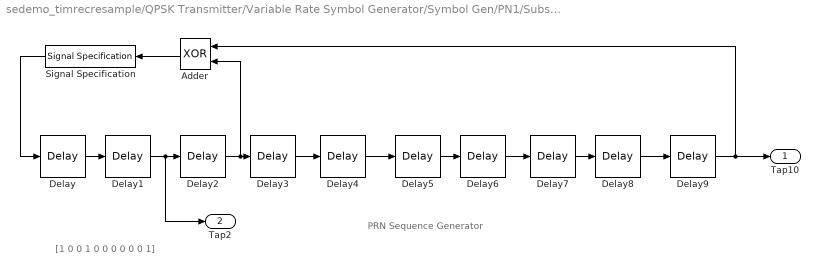
== system sedemo_timrecresample/QPSK Transmitter/Variable Rate Symbol Generator/Symbol Gen/PN1/Subsystem1 ==
  note: PRN Sequence Generator
  note: [1 0 0 1 0 0 0 0 0 0 1]
  Adder : Logic  Operator=XOR
  Delay{,1..5} (6 alike) : dspsigops/Delay  dly_unit=Samples  delay=1  ic_detail=on  dif_ic_for_ch=off  dif_ic_for_dly=off  ic=1  reset_popup=None
  Delay{6..9} (4 alike) : dspsigops/Delay  dly_unit=Samples  delay=1  ic_detail=on  dif_ic_for_ch=off  dif_ic_for_dly=off  ic=0  reset_popup=None
  Signal Specification : SignalSpecification  OutDataType=sfix(16)  OutScaling=2^0
  Tap10 : Outport  OutDataType=sfix(16)  OutScaling=2^0  InitialOutput=0
  Tap2 : Outport  Port=2  OutDataType=sfix(16)  OutScaling=2^0  InitialOutput=0
  wires:
  Signal Specification/1 -> Delay/1
  Delay9/1 -> Adder/1, Tap10/1
  Delay/1 -> Delay1/1
  Delay1/1 -> Delay2/1, Tap2/1
  Delay3/1 -> Delay4/1
  Delay4/1 -> Delay5/1
  Delay5/1 -> Delay6/1
  Delay6/1 -> Delay7/1
  Delay7/1 -> Delay8/1
  Delay8/1 -> Delay9/1
  Adder/1 -> Signal Specification/1
  Delay2/1 -> Delay3/1, Adder/2

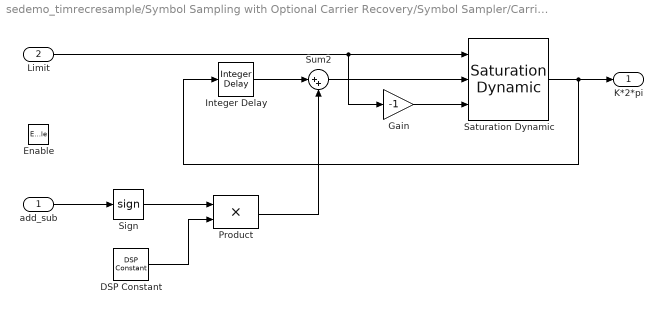
== system sedemo_timrecresample/Symbol Sampling with Optional Carrier Recovery/Symbol Sampler/Carrier Recovery/Limited Phase Unwrapper/N*2*pi accumulator ==
  add_sub : Inport  OutDataType=sfix(16)  OutScaling=2^0
  Limit : Inport  Port=2  OutDataType=sfix(16)  OutScaling=2^0
  Enable : EnablePort
  DSP Constant : dspsrcs4/DSP Constant  SystemSampleTime=-1  Value=-2*pi  SampleMode=Discrete  discreteOutput=Sample-based  continuousOutput=Sample-based  sampTime=inf  framePeriod=2  dataType=Inherit from 'Constant value'  isSigned=on  wordLen=16  udDataType=sfix(16)  fracBitsMode=Best precision  numFracBits=15  InterpretAs1D=-inf  Ts=-inf  FramebasedOutput=-inf
  Gain : Gain  Gain=-1  ParameterDataType=sfix(16)  ParameterScaling=2^0  OutDataType=sfix(16)  OutScaling=2^0
  Integer Delay : simulink/Discrete/Integer Delay  vinit=0.0  samptime=-1  NumDelays=1
  Product : Product  OutDataType=sfix(16)  OutScaling=2^0  SaturateOnIntegerOverflow=on  OutDataTypeStr=Inherit: Same as first input
  Saturation Dynamic : simulink/Discontinuities/Saturation Dynamic  SystemSampleTime=-1  OutMin=[]  OutMax=[]  OutDataTypeStr=Inherit: Same as second input  OutDataType=sfix(16)  OutScaling=2^-10  DoSatur=off
  Sign : Signum
  Sum2 : Sum  Inputs=|++  OutDataType=sfix(16)  OutScaling=2^0  SaturateOnIntegerOverflow=on
  K*2*pi : Outport  OutDataType=sfix(16)  OutScaling=2^0
  wires:
  Integer Delay/1 -> Sum2/1
  DSP Constant/1 -> Product/2
  Sign/1 -> Product/1
  Product/1 -> Sum2/2
  add_sub/1 -> Sign/1
  Sum2/1 -> Saturation Dynamic/2
  Saturation Dynamic/1 -> K*2*pi/1, Integer Delay/1
  Gain/1 -> Saturation Dynamic/3
  Limit/1 -> Gain/1, Saturation Dynamic/1

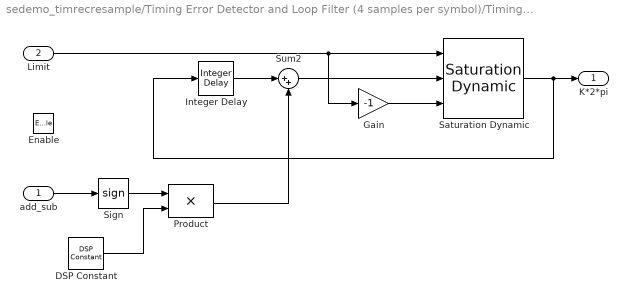
== system sedemo_timrecresample/Timing Error Detector and Loop Filter (4 samples per symbol)/Timing Error Detector/Timing Error/Limited Phase Unwrapper/N*2*pi accumulator ==
  add_sub : Inport  OutDataType=sfix(16)  OutScaling=2^0
  Limit : Inport  Port=2  OutDataType=sfix(16)  OutScaling=2^0
  Enable : EnablePort
  DSP Constant : dspsrcs4/DSP Constant  SystemSampleTime=-1  Value=-2*pi  SampleMode=Discrete  discreteOutput=Sample-based  continuousOutput=Sample-based  sampTime=inf  framePeriod=2  dataType=Inherit from 'Constant value'  isSigned=on  wordLen=16  udDataType=sfix(16)  fracBitsMode=Best precision  numFracBits=15  InterpretAs1D=-inf  Ts=-inf  FramebasedOutput=-inf
  Gain : Gain  Gain=-1  ParameterDataType=sfix(16)  ParameterScaling=2^0  OutDataType=sfix(16)  OutScaling=2^0
  Integer Delay : simulink/Discrete/Integer Delay  vinit=0.0  samptime=-1  NumDelays=1
  Product : Product  OutDataType=sfix(16)  OutScaling=2^0  SaturateOnIntegerOverflow=on  OutDataTypeStr=Inherit: Same as first input
  Saturation Dynamic : simulink/Discontinuities/Saturation Dynamic  SystemSampleTime=-1  OutMin=[]  OutMax=[]  OutDataTypeStr=Inherit: Same as second input  OutDataType=sfix(16)  OutScaling=2^-10  DoSatur=off
  Sign : Signum
  Sum2 : Sum  Inputs=|++  OutDataType=sfix(16)  OutScaling=2^0  SaturateOnIntegerOverflow=on
  K*2*pi : Outport  OutDataType=sfix(16)  OutScaling=2^0
  wires:
  Integer Delay/1 -> Sum2/1
  DSP Constant/1 -> Product/2
  Sign/1 -> Product/1
  Product/1 -> Sum2/2
  add_sub/1 -> Sign/1
  Sum2/1 -> Saturation Dynamic/2
  Saturation Dynamic/1 -> K*2*pi/1, Integer Delay/1
  Gain/1 -> Saturation Dynamic/3
  Limit/1 -> Gain/1, Saturation Dynamic/1
